simulink model "Multilevel_3ph"  (Simulink 8.1)
settings: Solver=ode23tb  StartTime=0.0  StopTime=0.08  MaxStep=1e-6  RelTol=1e-3
InitFcn:
  | R = 10
  | L = 10e-3
libraries: powerlib x27, simulink x3
settings Model: Creator=Elijah  LastModifiedBy=Elijah
settings DataIOCC: SignalLoggingSaveFormat=Dataset
settings OptimizationCC: ExpressionDepthLimit=128
settings DebuggingCC: FcnCallInpInsideContextMsg=EnableAllAsError
settings GRTTargetCC: CombineOutputUpdateFcns=on  GRTInterface=off

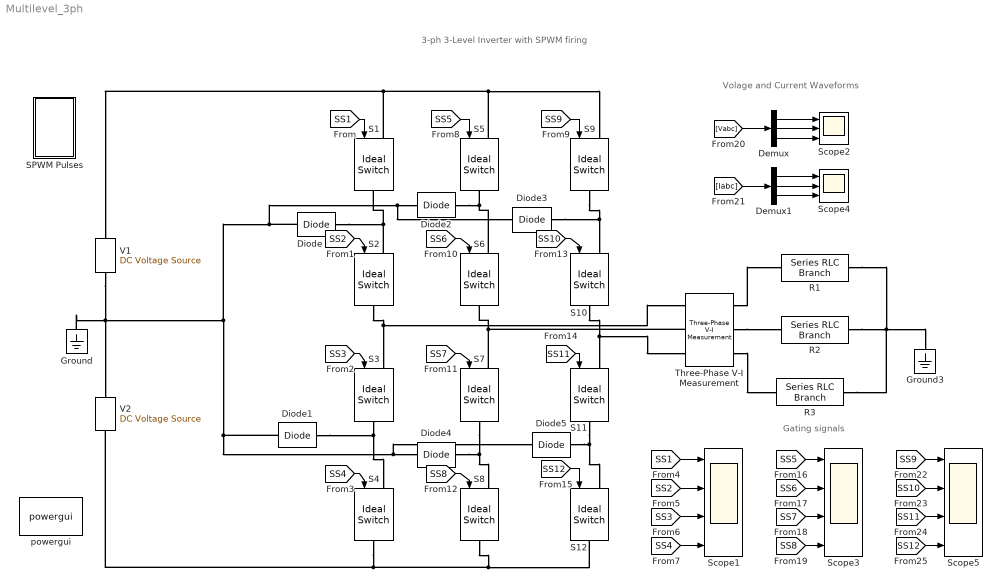
== system Multilevel_3ph ==
  note: Gating signals
  note: Volage and Current Waveforms
  note: 3-ph 3-Level Inverter with SPWM firing
  Demux : Demux  Outputs=3
  Demux1 : Demux  Outputs=3
  Diode{,1..5} (6 alike) : powerlib/Power Electronics/Diode  Ron=0.001  Lon=0  Vf=0.8  IC=0  UseSnubber=off  Rs=500  Cs=250e-9  Measurements=off
  Ground : powerlib/Elements/Ground  LConnTagsString=a
  Ground3 : powerlib/Elements/Ground  LConnTagsString=a
  R1 : powerlib/Elements/Series RLC Branch  LConnTagsString=__new0  RConnTagsString=__new0  BranchType=RL  Resistance=R  Inductance=L  SetiL0=off  InitialCurrent=0  Capacitance=1e-6  Setx0=off  InitialVoltage=0  Measurements=Branch voltage and current
  R2 : powerlib/Elements/Series RLC Branch  LConnTagsString=__new0  RConnTagsString=__new0  BranchType=RL  Resistance=R  Inductance=L  SetiL0=off  InitialCurrent=0  Capacitance=1e-6  Setx0=off  InitialVoltage=0  Measurements=Branch voltage and current
  R3 : powerlib/Elements/Series RLC Branch  LConnTagsString=__new0  RConnTagsString=__new0  BranchType=RL  Resistance=R  Inductance=L  SetiL0=off  InitialCurrent=0  Capacitance=1e-6  Setx0=off  InitialVoltage=0  Measurements=Branch voltage and current
  S{1..12} (12 alike) : powerlib/Power Electronics/Ideal Switch  Ron=0.001  Lon=0  IC=0  Rs=1e5  Cs=inf  Measurements=off
  SPWM Pulses : Subsystem  mask(Sine PWM for 3ph-3level Inverter){Ma=0.8, fr=50, Mf=21}
      mask prompts: Ma "Modulation Index"; fr "Reference Frequency"; Mf "Modulation Frequency"
      mask help:
      | This block gives the 12 pulses for a 3-ph 3-level inverter.
      | The parameters that you can change are:
      | 1) Modulation Index (Ma) : this controls the rms output voltage
      | 2) Reference Frequency (fr) : sets the output voltage frequency
      | 3) Modulation Frequency (Mf) : sets the carrier frequency as multiple of fr
      mask init:
      | Ma = 0.8;
      | fr = 50;
      | Mf = 21;
  Scope1 : Scope  NumInputPorts=4
      settings: YMin=-5~-5~-5~-5  YMax=5~5~5~5
  Scope2 : Scope  NumInputPorts=3
      settings: YMin=-200~-200~-200  YMax=200~200~200  SaveName=Vabc
  Scope3 : Scope  NumInputPorts=4
      settings: YMin=-5~-5~-5~-5  YMax=5~5~5~5  SaveName=ScopeData6
  Scope4 : Scope  NumInputPorts=3
      settings: TimeRange=0.08  YMin=-10~-10~-10  YMax=10~10~10  SaveName=Iabc
  Scope5 : Scope  NumInputPorts=4
      settings: YMin=-5~-5~-5~-5  YMax=5~5~5~5  SaveName=ScopeData8
  Three-Phase V-I Measurement : powerlib/Measurements/Three-Phase V-I Measurement  VoltageMeasurement=phase-to-phase  SetLabelV=on  LabelV=Vabc  Vpu=off  VpuLL=off  CurrentMeasurement=yes  SetLabelI=on  LabelI=Iabc  Ipu=off  Pbase=100e6  Vbase=500e3  OutputType=Complex  PhasorSimulation=off  PSBequivalent=0
  V1 : powerlib/Electrical Sources/DC Voltage Source  Amplitude=100  Measurements=None
  V2 : powerlib/Electrical Sources/DC Voltage Source  Amplitude=100  Measurements=None
  powergui : powerlib/powergui  Priority=1  SimulationMode=Continuous  SolverType=Tustin  SampleTime=50e-6  frequency=60  SPID=off  DisableSnubberDevices=off  DisableRonSwitches=off  DisableVfSwitches=off  SwTol=0  Interpol=off  DisplayEquations=off  frequencyindice=0  Pbase=100e6  ErrMax=1e-4  Iterations=50  UnitsV=kV  UnitsW=MW  FunctionMessages=off  echomessages=off  HookPort=off  EnableUseOfTLC=off  x0status=blocks  RestoreLinks=warning  ResistiveCurrentMeasurement=off  Frange=[0:2:500]  Ylog=off  Xlog=on  ShowGrid=off  save=off  variable=ZData  structure=Vabc  ZoomFFT=off  StartTime=0.02  cycles=1  DisplayStyle=1  fundamental=50  FreqAxis=on  MaxFrequency=5000  frequencyindicesteady=1  RmsSteady=1  display=off  Ts=0  methode=off
  wires:
  [SS2] -> S2/1
  [SS1] -> S1/1
  [SS3] -> S3/1
  [SS4] -> S4/1
  [SS1] -> Scope1/1
  [SS2] -> Scope1/2
  [SS3] -> Scope1/3
  [SS4] -> Scope1/4
  [SS5] -> S5/1
  [SS9] -> S9/1
  [SS6] -> S6/1
  [SS7] -> S7/1
  [SS8] -> S8/1
  [SS10] -> S10/1
  [SS11] -> S11/1
  [SS12] -> S12/1
  [SS5] -> Scope3/1
  [SS6] -> Scope3/2
  [SS7] -> Scope3/3
  [SS8] -> Scope3/4
  [Vabc] -> Demux/1
  Demux/3 -> Scope2/3
  Demux/1 -> Scope2/1
  Demux/2 -> Scope2/2
  [Iabc] -> Demux1/1
  Demux1/3 -> Scope4/3
  Demux1/1 -> Scope4/1
  Demux1/2 -> Scope4/2
  [SS9] -> Scope5/1
  [SS10] -> Scope5/2
  [SS11] -> Scope5/3
  [SS12] -> Scope5/4
  connections:
  S5/LConn1 -- S1/LConn1 -- V1/RConn1 -- S9/LConn1
  S8/RConn1 -- S12/RConn1 -- S4/RConn1 -- V2/LConn1
  S2/RConn1 -- Three-Phase V-I Measurement/LConn1 -- S3/LConn1
  S3/RConn1 -- S4/LConn1 -- Diode1/LConn1
  S2/LConn1 -- Diode/RConn1 -- S1/RConn1
  V1/LConn1 -- Ground/LConn1 -- Diode/LConn1 -- Diode3/LConn1 -- Diode2/LConn1 -- Diode1/RConn1 -- Diode5/RConn1 -- Diode4/RConn1 -- V2/RConn1
  S7/RConn1 -- S8/LConn1 -- Diode4/LConn1
  S7/LConn1 -- Three-Phase V-I Measurement/LConn2 -- S6/RConn1
  S6/LConn1 -- Diode2/RConn1 -- S5/RConn1
  S9/RConn1 -- S10/LConn1 -- Diode3/RConn1
  S10/RConn1 -- S11/LConn1 -- Three-Phase V-I Measurement/LConn3
  S11/RConn1 -- Diode5/LConn1 -- S12/LConn1
  R2/RConn1 -- R3/RConn1 -- Ground3/LConn1 -- R1/RConn1
  Three-Phase V-I Measurement/RConn2 -- R2/LConn1
  Three-Phase V-I Measurement/RConn1 -- R1/LConn1
  Three-Phase V-I Measurement/RConn3 -- R3/LConn1

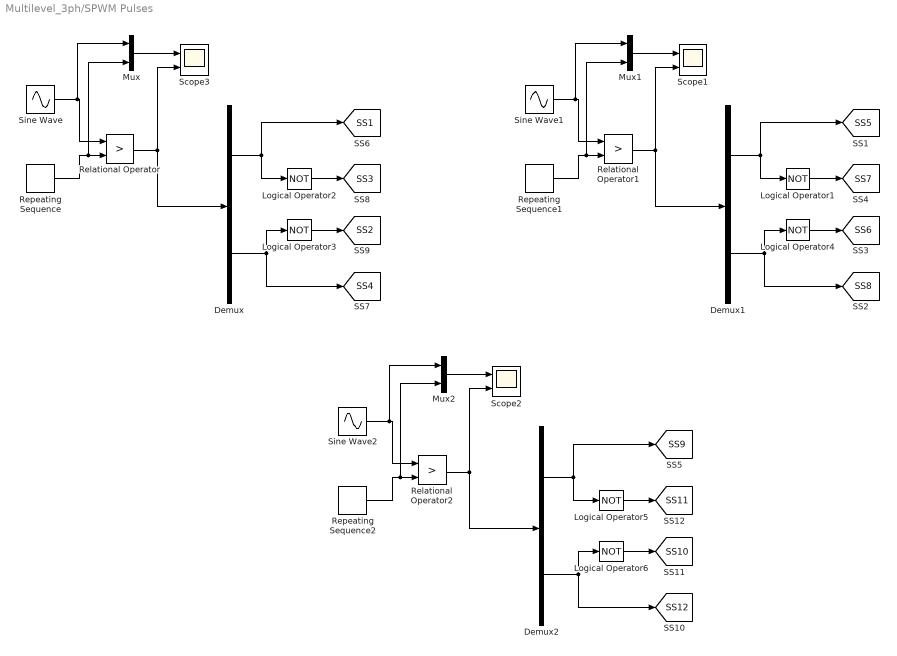
== system Multilevel_3ph/SPWM Pulses ==
  Demux : Demux  Outputs=2
  Demux1 : Demux  Outputs=2
  Demux2 : Demux  Outputs=2
  Logical Operator{1..6} (6 alike) : Logic  Operator=NOT  AllPortsSameDT=off  OutDataTypeStr=boolean
  Mux : Mux  Inputs=2
  Mux1 : Mux  Inputs=2
  Mux2 : Mux  Inputs=2
  Relational Operator : RelationalOperator  Operator=>  OutDataTypeStr=boolean
  Relational Operator1 : RelationalOperator  Operator=>  OutDataTypeStr=boolean
  Relational Operator2 : RelationalOperator  Operator=>  OutDataTypeStr=boolean
  Repeating Sequence : simulink/Sources/Repeating Sequence  rep_seq_t=[0 0.5 1]*(1/fr)*(1/Mf)*(1/2)  rep_seq_y=[0 1 0]
  Repeating Sequence1 : simulink/Sources/Repeating Sequence  rep_seq_t=[0 0.5 1]*(1/fr)*(1/Mf)*(1/2)  rep_seq_y=[0 1 0]
  Repeating Sequence2 : simulink/Sources/Repeating Sequence  rep_seq_t=[0 0.5 1]*(1/fr)*(1/Mf)*(1/2)  rep_seq_y=[0 1 0]
  Scope1 : Scope  NumInputPorts=2
      settings: YMin=-5~-5  YMax=5~5  SaveName=ScopeData2
  Scope2 : Scope  NumInputPorts=2
      settings: YMin=-5~-5  YMax=5~5  SaveName=ScopeData4
  Scope3 : Scope  NumInputPorts=2
      settings: YMin=-5~-5  YMax=5~5  SaveName=ScopeData3
  Sine Wave : Sin  Amplitude=Ma  Frequency=2*pi*fr  Phase=[0 pi]  SampleTime=0
  Sine Wave1 : Sin  Amplitude=Ma  Frequency=2*pi*fr  Phase=[0 pi] - 2*pi/3  SampleTime=0
  Sine Wave2 : Sin  Amplitude=Ma  Frequency=2*pi*fr  Phase=[0 pi] + 2*pi/3  SampleTime=0
  tag scope: SS10=global, SS11=global, SS12=global, SS1=global, SS2=global, SS3=global, SS4=global, SS5=global, SS6=global, SS7=global, SS8=global, SS9=global
  wires:
  Demux/2 -> Logical Operator3/1, [SS4]
  Mux/1 -> Scope3/1
  Repeating Sequence/1 -> Mux/2, Relational Operator/2
  Relational Operator/1 -> Demux/1, Scope3/2
  Sine Wave/1 -> Mux/1, Relational Operator/1
  Demux/1 -> Logical Operator2/1, [SS1]
  Logical Operator2/1 -> [SS3]
  Logical Operator3/1 -> [SS2]
  Demux1/2 -> [SS8], Logical Operator4/1
  Mux1/1 -> Scope1/1
  Repeating Sequence1/1 -> Relational Operator1/2, Mux1/2
  Relational Operator1/1 -> Scope1/2, Demux1/1
  Sine Wave1/1 -> Relational Operator1/1, Mux1/1
  Demux1/1 -> [SS5], Logical Operator1/1
  Demux2/2 -> Logical Operator6/1, [SS12]
  Mux2/1 -> Scope2/1
  Repeating Sequence2/1 -> Mux2/2, Relational Operator2/2
  Relational Operator2/1 -> Demux2/1, Scope2/2
  Sine Wave2/1 -> Mux2/1, Relational Operator2/1
  Demux2/1 -> Logical Operator5/1, [SS9]
  Logical Operator1/1 -> [SS7]
  Logical Operator4/1 -> [SS6]
  Logical Operator5/1 -> [SS11]
  Logical Operator6/1 -> [SS10]
